simulink model "LoggerFile"  (R2024a)
settings: Solver=VariableStepAuto  StartTime=0.0  StopTime=10.0  RelTol=1e-3
undefined symbols (not defined in the file or in its folder): canChannel
libraries: canmsglib x3, canlib x2
settings Model: DataDictionary=BMS_System_dict1.sldd  Creator=hirah  LastModifiedBy=hirah

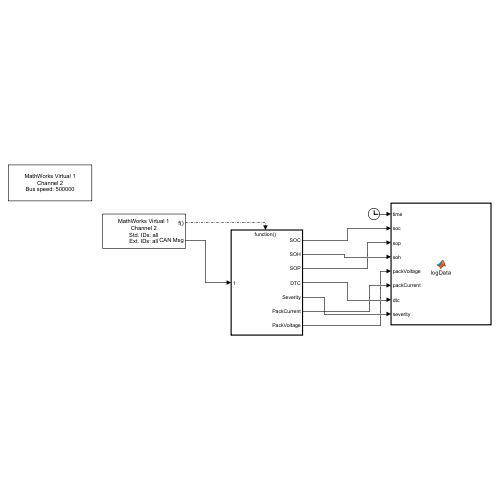
[thumbnail: Simulink's stored preview of the top-level diagram]
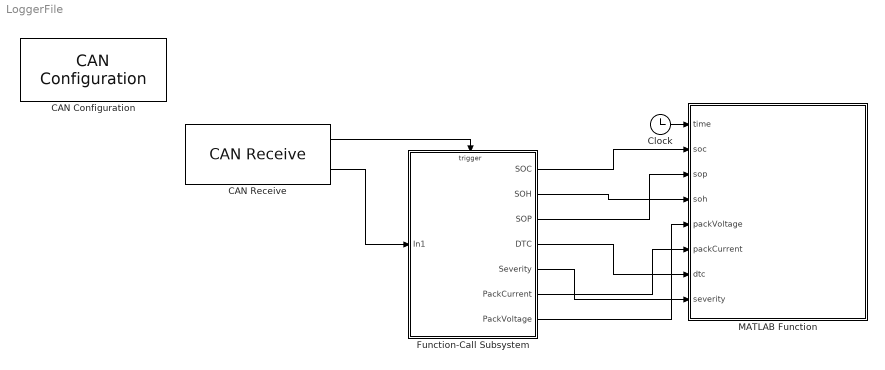
== system LoggerFile ==
  CAN Configuration : canlib/CAN Configuration  BlockHandle=570.0001  Device=MathWorks Virtual 1 (Channel 2)  DeviceMenu=MathWorks Virtual 1 (Channel 2)  ObjConstructor=canChannel('MathWorks', 'Virtual 1', 2)  BusSpeed=500000  EnableBitParameters=off  AckMode=Normal
  CAN Receive : canlib/CAN Receive  BlockHandle=729.0002  Device=MathWorks Virtual 1 (Channel 2)  DeviceMenu=MathWorks Virtual 1 (Channel 2)  ObjConstructor=canChannel('MathWorks', 'Virtual 1', 2)  EnableStandardIDsFilter=off  StdIDsCombo=Allow all  StandardIDs=261  EnableExtendedIDsFilter=off  ExtIDsCombo=Allow all  ExtendedIDs=0  SampleTime=0.01  MsgsPerTimestep=all  InternalFilterUpdateStatus=on  BusOutput=off
  Clock : Clock
  Function-Call Subsystem : Subsystem  TreatAsAtomicUnit=on
  MATLAB Function : MATLAB Function  TreatAsAtomicUnit=on
  wires:
  Clock/1 -> MATLAB Function/1(time)
  CAN Receive/2 -> Function-Call Subsystem/1(In1)
  CAN Receive/1 -> Function-Call Subsystem/Trigger
  Function-Call Subsystem/1(SOC) -> MATLAB Function/2(soc)
  Function-Call Subsystem/2(SOH) -> MATLAB Function/4(soh)
  Function-Call Subsystem/3(SOP) -> MATLAB Function/3(sop)
  Function-Call Subsystem/4(DTC) -> MATLAB Function/7(dtc)
  Function-Call Subsystem/5(Severity) -> MATLAB Function/8(severity)
  Function-Call Subsystem/6(PackCurrent) -> MATLAB Function/6(packCurrent)
  Function-Call Subsystem/7(PackVoltage) -> MATLAB Function/5(packVoltage)

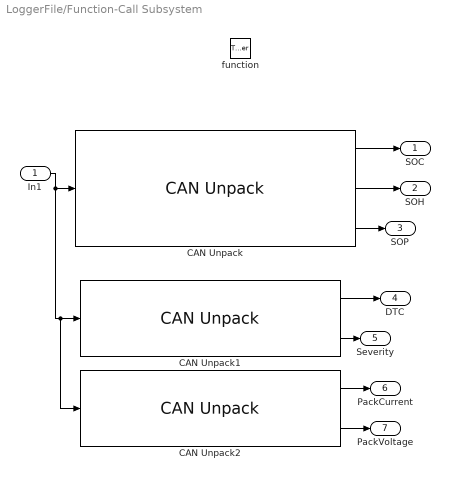
== system LoggerFile/Function-Call Subsystem ==
  In1 : Inport
  function : TriggerPort  TriggerType=function-call  VariantControl=(inherit)
  CAN Unpack : canmsglib/CAN Unpack  CANdbFile=C:\Users\hirah\Downloads\BMS_CAN_Database (5).dbc  MsgList=frmBMSStateEstimation  MsgName=frmBMSStateEstimation  MsgIDType=Standard (11-bit identifier)  MsgIdentifier=259  MsgLength=6  SignalInfo={ 'sigSOC', '0', '8', 'LE', 'unsigned', 'Standard', '0', '1', '0', '0', '100'; 'sigSOH', '8', '8', 'LE', 'unsigned', 'Standard', '0', '1', '0', '0', '100'; 'sigSOPCharge', '32', '16', 'LE', 'unsigned', 'Standard', '0', '1', '0', '0', '200' }  IDPort=off  TimestampPort=off  ErrorPort=off  RemotePort=off  LengthPort=off  StatusPort=off  ApplyMinMax=off
  CAN Unpack1 : canmsglib/CAN Unpack  CANdbFile=C:\Users\hirah\Downloads\BMS_CAN_Database (5).dbc  MsgList=frmDiagnosticDTC  MsgName=frmDiagnosticDTC  MsgIDType=Standard (11-bit identifier)  MsgIdentifier=264  MsgLength=3  SignalInfo={'sigDTCCode1','0','16','LE','unsigned','Standard','0','1','0','0','65535';'sigDTCSeverity1','16','8','LE','unsigned','Standard','0','1','0','0','3'}  IDPort=off  TimestampPort=off  ErrorPort=off  RemotePort=off  LengthPort=off  StatusPort=off  ApplyMinMax=off
      settings: DataFormat=CANdb specified signals
  CAN Unpack2 : canmsglib/CAN Unpack  CANdbFile=C:\Users\hirah\Downloads\BMS_CAN_Database (5).dbc  MsgList=frmPackMeasurements  MsgName=frmPackMeasurements  MsgIDType=Standard (11-bit identifier)  MsgIdentifier=256  MsgLength=6  SignalInfo={ 'sigPackCurrent', '16', '16', 'LE', 'signed', 'Standard', '0', '0.1', '0', '-400', '400'; 'sigPackVoltage', '0', '16', 'LE', 'unsigned', 'Standard', '0', '0.1', '0', '0', '1000' }  IDPort=off  TimestampPort=off  ErrorPort=off  RemotePort=off  LengthPort=off  StatusPort=off  ApplyMinMax=off
  SOC : Outport
  SOH : Outport  Port=2
  SOP : Outport  Port=3
  DTC : Outport  Port=4
  Severity : Outport  Port=5
  PackCurrent : Outport  Port=6
  PackVoltage : Outport  Port=7
  wires:
  In1/1 -> CAN Unpack2/1, CAN Unpack1/1, CAN Unpack/1
  CAN Unpack/1 -> SOC/1
  CAN Unpack/2 -> SOH/1
  CAN Unpack/3 -> SOP/1
  CAN Unpack1/1 -> DTC/1
  CAN Unpack1/2 -> Severity/1
  CAN Unpack2/1 -> PackCurrent/1
  CAN Unpack2/2 -> PackVoltage/1

== matlab function LoggerFile/MATLAB Function ==
  data: time input; soc input; sop input; soh input; packVoltage input; packCurrent input; dtc input; severity input
function logData(time, soc, sop, soh, packVoltage, packCurrent, dtc,severity)
    if nargin ~= 7
        error('8 inputs required: time, soc, sop, soh, packVoltage, packCurrent, dtc,severity');
    end
    filename = 'bms_log.csv';
    fileExists = isfile(filename);
    fid = fopen(filename, 'a');
    if ~fileExists
        fprintf(fid, 'Time,SOC,SOP,SOH,PackVoltage,PackCurrent,DTC,severity\n');
    end
    fprintf(fid, '%.3f,%.2f,%.2f,%.2f,%.2f,%.2f,%s,%s\n', ...
        time, soc, sop, soh, packVoltage, packCurrent, string(dtc),string(severity));
    fclose(fid);
end
